simulink model "MIL4L3_SW6_V1_20220211"  (R2018b)
settings: Solver=FixedStepAuto  StartTime=0.0  StopTime=inf  FixedStep=0.001  RelTol=1e-3
PreLoadFcn:
  | A0_MILtest;
undefined symbols (not defined in the file or in its folder): Clb_ICADirect_LaneDisp_StateFive, Clb_ICADirect_LaneDisp_StateFour, Clb_ICADirect_LaneDisp_StateOne, Clb_ICADirect_LaneDisp_StateThree, Clb_ICADirect_LaneDisp_StateTwo, Clb_ICADirect_LaneDisp_StateZero, Clb_ICADirect_LaneDispSW, Clb_ICADirect_TrnLghtsCom_Switch, Clb_ICADirect_TrnLghtsCom_Value, Clb_ICADirect_TrnLghtsCrtl_Inhb, IMAP_Clb_ACU_Driver_Belt, IMAP_Clb_ACU_Driver_Belt_Over, IMAP_Clb_ACU_Passenger_Belt, IMAP_Clb_ACU_Passenger_Belt_Over, IMAP_Clb_ACU_RearLeft_Belt, IMAP_Clb_ACU_RearLeft_Belt_Over, IMAP_Clb_ACU_RearMiddle_Belt, IMAP_Clb_ACU_RearMiddle_Belt_Over, IMAP_Clb_ACU_RearRight_Belt, IMAP_Clb_ACU_RearRight_Belt_Over, IMAP_Clb_AEB_Switch, IMAP_Clb_AEB_Switch_Over, IMAP_Clb_ALC_TLC_Mode, IMAP_Clb_ALC_TLC_Mode_Over, IMAP_Clb_BCM_Battery_Voltage, IMAP_Clb_BCM_Battery_Voltage_Over, IMAP_Clb_BCM_BrakeLamp_State, IMAP_Clb_BCM_BrakeLamp_State_Over, IMAP_Clb_BCM_CHMSL_Status, IMAP_Clb_BCM_CHMSL_Status_Over, IMAP_Clb_BCM_Door_Lock_State, IMAP_Clb_BCM_Door_Lock_State_Over, IMAP_Clb_BCM_FrontWiper_State, IMAP_Clb_BCM_FrontWiper_State_Over, IMAP_Clb_BCM_FrontWiper_Switch, IMAP_Clb_BCM_FrontWiper_Switch_Over, IMAP_Clb_BCM_HazardLamp, IMAP_Clb_BCM_HazardLamp_Over, IMAP_Clb_BCM_HazardLamp_Switch, IMAP_Clb_BCM_HazardLamp_Switch_Over, IMAP_Clb_BCM_HighBeam_State, IMAP_Clb_BCM_HighBeam_State_Over, IMAP_Clb_BCM_Ignition_State, IMAP_Clb_BCM_Ignition_State_Over, IMAP_Clb_BCM_IHBC_Enabled, IMAP_Clb_BCM_IHBC_Enabled_Over, IMAP_Clb_BCM_Left_Light, IMAP_Clb_BCM_Left_Light_Over, IMAP_Clb_BCM_LeftTurn_Switch, IMAP_Clb_BCM_LeftTurn_Switch_Over, IMAP_Clb_BCM_LF_Door_State, IMAP_Clb_BCM_LF_Door_State_Over, IMAP_Clb_BCM_LowBeam_State, IMAP_Clb_BCM_LowBeam_State_Over, IMAP_Clb_BCM_LR_Door_State, IMAP_Clb_BCM_LR_Door_State_Over, IMAP_Clb_BCM_RF_Door_State, IMAP_Clb_BCM_RF_Door_State_Over, IMAP_Clb_BCM_Right_Light, IMAP_Clb_BCM_Right_Light_Over ... (+547)
libraries: CarMaker4SL x2153, simulink x292, dspstat3 x3, canmsglib x2, simulink_extras x1
(part 13 of 52)

== system MIL4L3_SW6_V1_20220211/CarMaker/VehicleControl/FunctionDataLog/ICA ==
  Bus Selector : BusSelector  OutputSignals=FDMMve_d_IcaFcnConf,FDMMve_d_SignalTStamp
  Bus Selector1 : BusSelector  OutputSignals=IMAPve_d_RCTA_Swtich,IMAPve_d_DOW_Switch,IMAPve_d_JA_Brake_Switch,IMAPve_d_JA_Alert_Switch,IMAPve_d_EPS_LKA_State,IMAPve_d_EPS_Trq_State,IMAPve_d_SAS_Clb_State,IMAPve_d_SAS_Trim_State,IMAPve_d_EPS_TrqLim_State,IMAPve_g_ESC_LatAcc,IMAPve_d_ESC_LatAcc_Valid,IMAPve_g_ESC_YawRate,IMAPve_g_ESC_VehSpd,IMAPve_g_ESC_LonAcc,IMAPve_d_ESC_LonAcc_Valid,IMAPve_g_ESC_Brake_Press,IMAPve_g_ESC_Static_Slope,IMAPve_g_ESC_DySlope_Accuracy,IMAPve_g_ESC_DySlope,IMAPve_g_SW_Angle_Speed,IMAPve_d_BCM_Trunk_State,IMAPve_d_PEPS_Door_Lock_Req,IMAPve_g_EMS_MinTWhl_Offset,IMAPve_g_EMS_ACC_VirtualPedal,IMAPve_d_EMS_AccPedal_Fault,IMAPve_d_ESC_Veh_Standstill,IMAPve_d_TCU_Actual_Gear,IMAPve_d_BCM_Ignition_State,IMAPve_d_SWS_Failure_Status,IMAPve_d_ESC_OFF,IMAPve_d_ESC_AlarmSig,IMAPve_d_ESC_RR_Wheel_Pulse,IMAPve_d_ESC_AEB_Available,IMAPve_d_ESC_ACC_Active,IMAPve_d_BCM_CHMSL_Status,IMAPve_d_BCM_BrakeLamp_State,IMAPve_d_ACU_Passenger_Belt,IMAPve_d_EPB_Warn_Req,IMAPve_d_EPB_Switch_State,IMAPve_d_ESC_Hold_State,IMAPva_g_ORI_Obj_LongDis,IMAPva_g_ORI_Obj_LAngle,IMAPva_g_ORI_Obj_RAngle,IMAPva_g_ORI_Obj_Width,IMAPva_d_ORI_Obj_ID,IMAPve_g_ORI_L0_C3,IMAPve_g_ORI_L0_C2,IMAPve_g_ORI_L0_C1,IMAPve_g_ORI_L0_C0,IMAPve_d_ORI_L0_Type,IMAPve_g_ORI_L0_VR,IMAPve_g_ORI_L0_W,IMAPve_g_ORI_L1_C3,IMAPve_g_ORI_L1_C2,IMAPve_g_ORI_L1_C1,IMAPve_g_ORI_L1_C0,IMAPve_d_ORI_L1_Type,IMAPve_g_ORI_L1_VR,IMAPve_g_ORI_L1_W,IMAPve_g_ORI_R0_C3,IMAPve_g_ORI_R0_C2,IMAPve_g_ORI_R0_C1,IMAPve_g_ORI_R0_C0,IMAPve_d_ORI_R0_LT,IMAPve_g_ORI_R0_VR,IMAPve_g_ORI_R0_W,IMAPve_g_ORI_R1_C3,IMAPve_g_ORI_R1_C2,IMAPve_d_Sensor_Status,IMAPve_d_RF_Radar_Status,IMAPve_d_LR_Radar_Status,IMAPve_d_RR_Radar_Status,IMAPve_d_Fusion_Status,IMAPve_d_Fusion_Time_Stamp,IMAPve_d_obj_Num,IMAPva_d_obj_id,IMAPva_g_obj_pos_x,IMAPva_g_obj_pos_y,IMAPva_g_obj_vel_x,IMAPva_g_obj_vel_y,IMAPva_g_obj_acc_x,IMAPva_g_obj_acc_y,IMAPva_g_obj_pos_var_x,IMAPva_g_obj_pos_var_y,IMAPva_g_obj_pos_var_xy,IMAPva_g_obj_width,IMAPva_g_obj_length,IMAPva_d_obj_class,IMAPva_d_obj_lane,IMAPva_d_obj_status,IMAPva_d_obj_age,IMAPva_d_obj_TurnLight,IMAPva_d_obj_BrakeLight,IMAPva_d_obj_MotionStatus,IMAPve_d_Road_Type,IMAPve_g_L0_C0,IMAPve_g_L0_C1,IMAPve_g_L0_C2,IMAPve_g_L0_C3,IMAPve_g_L0_VR,IMAPve_d_L0_Q,IMAPve_d_L0_Type,IMAPve_g_L0_W,IMAPve_g_R0_C0,IMAPve_g_R0_C1,IMAPve_g_R0_C2,IMAPve_g_R0_C3,IMAPve_g_R0_VR,IMAPve_d_R0_Q,IMAPve_d_R0_Type,IMAPve_g_R0_W,IMAPve_g_L1_C0,IMAPve_g_L1_C1,IMAPve_g_L1_C2,IMAPve_g_L1_C3,IMAPve_g_L1_VR,IMAPve_d_L1_Q,IMAPve_d_L1_Type,IMAPve_g_L1_W,IMAPve_g_R1_C0,IMAPve_g_R1_C1,IMAPve_g_R1_C2,IMAPve_g_R1_C3,IMAPve_g_R1_VR,IMAPve_d_R1_Q,IMAPve_d_R1_Type,IMAPve_g_R1_W,IMAPve_g_L0_C0_Back,IMAPve_g_L0_C1_Back,IMAPve_g_L0_C2_Back,IMAPve_g_L0_C3_Back,IMAPve_g_L0_Range_Back,IMAPve_g_R0_C0_Back,IMAPve_g_R0_C1_Back,IMAPve_g_R0_C2_Back,IMAPve_g_R0_C3_Back,IMAPve_g_R0_Range_Back,IMAPve_g_L1_C0_Back,IMAPve_g_L1_C1_Back,IMAPve_g_L1_C2_Back,IMAPve_g_L1_C3_Back,IMAPve_g_L1_Range_Back,IMAPve_d_APA_AutoPark_WorkSt
  Bus Selector4 : BusSelector  OutputSignals=IMAPve_d_BCM_RF_Door_State,IMAPve_d_TSR_Sign_Type,IMAPve_g_Camera_Signal_Fault
  BusCreator2 : BusCreator  Inputs=158
  Clock1 : Clock
  Constant : Constant  Value=0  OutDataTypeStr=uint32
  Constant1 : Constant  Value=0  OutDataTypeStr=uint32
  Constant2 : Constant  Value=0  OutDataTypeStr=uint16
  Constant3 : Constant  OutDataTypeStr=uint8
  Constant4 : Constant  Value=0  OutDataTypeStr=uint8
  Constant5 : Constant  OutDataTypeStr=uint8
  Constant6 : Constant  Value=0  OutDataTypeStr=uint8
  Data Type Conversion{5..8} (4 alike) : DataTypeConversion
  Read CM Dict4 : CarMaker4SL/Read CM Dict  xname=User.IO.Out.VR_RR  xsync=off
  Read CM Dict5 : CarMaker4SL/Read CM Dict  xname=User.IO.Out.VR_R  xsync=off
  Read CM Dict6 : CarMaker4SL/Read CM Dict  xname=User.IO.Out.VR_LL  xsync=off
  Read CM Dict7 : CarMaker4SL/Read CM Dict  xname=User.IO.Out.VR_L  xsync=off
  Switch{4..7} (4 alike) : Switch  Threshold=20
  To Workspace : ToWorkspace  VariableName=ICABIn  SaveFormat=Timeseries  SampleTime=-1
  wires:
  Switch7/1 -> BusCreator2/100  "IMAPve_g_L0_VR"
  [ACCSva_d_ACCS2ICAB] -> BusCreator2/2  "ACCSva_d_ACCS2ICA"
  [EPS_LKA_State_ica] -> BusCreator2/5  "EPS_LKA_State"
  Clock1/1 -> BusCreator2/1  "System_Clock"
  BusCreator2/1 -> To Workspace/1
  Constant1/1 -> BusCreator2/150  "ADIAve_g_BSWFaultStatus"
  Constant/1 -> BusCreator2/149  "ADIAve_g_ASWFaultStatus"
  Constant3/1 -> BusCreator2/152  "EWWWve_y_BSD_LCWWorkingSt"
  Constant2/1 -> BusCreator2/151  "ADIAve_d_FuncFaultStatus"
  Constant6/1 -> BusCreator2/155  "EWWWve_y_BSD_S_LCAWarning"
  Constant4/1 -> BusCreator2/153  "EWWWve_y_BSD_LCAWarning"
  Constant5/1 -> BusCreator2/154  "EWWWve_y_BSD_S_LCWWorkingSt"
  Bus Selector4/2 -> BusCreator2/157  "<IMAPve_d_TSR_Sign_Type>"
  Bus Selector4/1 -> BusCreator2/156  "<IMAPve_d_BCM_RF_Door_State>"
  Bus Selector4/3 -> BusCreator2/158  "<IMAPve_g_Camera_Signal_Fault>"
  [IMAP_Output] -> Bus Selector1/1, Bus Selector4/1
  Read CM Dict4/1 -> Data Type Conversion8/1
  Bus Selector1/15 -> BusCreator2/20  "<IMAPve_d_ESC_LonAcc_Valid>"
  Bus Selector1/2 -> BusCreator2/7  "<IMAPve_d_DOW_Switch>"
  Bus Selector1/16 -> BusCreator2/21  "<IMAPve_g_ESC_Brake_Press>"
  Bus Selector1/9 -> BusCreator2/14  "<IMAPve_d_EPS_TrqLim_State>"
  Bus Selector1/11 -> BusCreator2/16  "<IMAPve_d_ESC_LatAcc_Valid>"
  Bus Selector1/13 -> BusCreator2/18  "<IMAPve_g_ESC_VehSpd>"
  Switch5/1 -> BusCreator2/108  "IMAPve_g_R0_VR"
  Bus Selector1/7 -> BusCreator2/12  "<IMAPve_d_SAS_Clb_State>"
  Bus Selector1/5 -> BusCreator2/10  "<IMAPve_d_EPS_LKA_State>"
  Bus Selector1/92 -> BusCreator2/97  "<IMAPva_d_obj_TurnLight>"
  Bus Selector1/52 -> BusCreator2/57  "<IMAPve_g_ORI_L0_W>"
  Bus Selector1/140 -> BusCreator2/145  "<IMAPve_g_L1_C2_Back>"
  Bus Selector1/62 -> BusCreator2/67  "<IMAPve_g_ORI_R0_C1>"
  Bus Selector1/115 -> BusCreator2/120  "<IMAPve_g_L1_C3>"
  Bus Selector1/87 -> BusCreator2/92  "<IMAPva_g_obj_length>"
  Bus Selector1/139 -> BusCreator2/144  "<IMAPve_g_L1_C1_Back>"
  Bus Selector1/22 -> BusCreator2/27  "<IMAPve_d_PEPS_Door_Lock_Req>"
  Bus Selector1/136 -> BusCreator2/141  "<IMAPve_g_R0_C3_Back>"
  Bus Selector1/132 -> BusCreator2/137  "<IMAPve_g_L0_Range_Back>"
  Bus Selector1/73 -> BusCreator2/78  "<IMAPve_d_Fusion_Status>"
  Bus Selector1/124 -> BusCreator2/129  "<IMAPve_g_R1_VR>"
  Bus Selector1/38 -> BusCreator2/43  "<IMAPve_d_EPB_Warn_Req>"
  Bus Selector1/122 -> BusCreator2/127  "<IMAPve_g_R1_C2>"
  Bus Selector1/105 -> BusCreator2/110  "<IMAPve_g_R0_C1>"
  Bus Selector1/137 -> BusCreator2/142  "<IMAPve_g_R0_Range_Back>"
  Bus Selector1/34 -> BusCreator2/39  "<IMAPve_d_ESC_ACC_Active>"
  Bus Selector1/133 -> BusCreator2/138  "<IMAPve_g_R0_C0_Back>"
  Bus Selector1/129 -> BusCreator2/134  "<IMAPve_g_L0_C1_Back>"
  Bus Selector1/109 -> BusCreator2/114  "<IMAPve_d_R0_Q>"
  Bus Selector1/126 -> BusCreator2/131  "<IMAPve_d_R1_Type>"
  Bus Selector1/56 -> BusCreator2/61  "<IMAPve_g_ORI_L1_C0>"
  Bus Selector1/106 -> BusCreator2/111  "<IMAPve_g_R0_C2>"
  Bus Selector1/93 -> BusCreator2/98  "<IMAPva_d_obj_BrakeLight>"
  Bus Selector1/127 -> BusCreator2/132  "<IMAPve_g_R1_W>"
  Bus Selector1/125 -> BusCreator2/130  "<IMAPve_d_R1_Q>"
  Bus Selector1/123 -> BusCreator2/128  "<IMAPve_g_R1_C3>"
  Bus Selector1/96 -> BusCreator2/101  "<IMAPve_g_L0_C0>"
  Bus Selector1/29 -> BusCreator2/34  "<IMAPve_d_SWS_Failure_Status>"
  Bus Selector1/114 -> BusCreator2/119  "<IMAPve_g_L1_C2>"
  Switch4/1 -> BusCreator2/124  "IMAPve_g_R1_VR"
  Bus Selector1/118 -> BusCreator2/123  "<IMAPve_d_L1_Type>"
  Bus Selector1/97 -> BusCreator2/102  "<IMAPve_g_L0_C1>"
  Bus Selector1/121 -> BusCreator2/126  "<IMAPve_g_R1_C1>"
  Bus Selector1/82 -> BusCreator2/87  "<IMAPva_g_obj_acc_y>"
  Bus Selector1/110 -> BusCreator2/115  "<IMAPve_d_R0_Type>"
  Bus Selector1/113 -> BusCreator2/118  "<IMAPve_g_L1_C1>"
  Bus Selector1/45 -> BusCreator2/50  "<IMAPva_d_ORI_Obj_ID>"
  Bus Selector1/80 -> BusCreator2/85  "<IMAPva_g_obj_vel_y>"
  Bus Selector1/24 -> BusCreator2/29  "<IMAPve_g_EMS_ACC_VirtualPedal>"
  Bus Selector1/117 -> BusCreator2/122  "<IMAPve_d_L1_Q>"
  Bus Selector1/128 -> BusCreator2/133  "<IMAPve_g_L0_C0_Back>"
  Bus Selector1/108 -> BusCreator2/113  "<IMAPve_g_R0_VR>"
  Bus Selector1/112 -> BusCreator2/117  "<IMAPve_g_L1_C0>"
  Bus Selector1/99 -> BusCreator2/104  "<IMAPve_g_L0_C3>"
  Bus Selector1/100 -> BusCreator2/105  "<IMAPve_g_L0_VR>"
  Bus Selector1/107 -> BusCreator2/112  "<IMAPve_g_R0_C3>"
  Bus Selector1/88 -> BusCreator2/93  "<IMAPva_d_obj_class>"
  Bus Selector1/102 -> BusCreator2/107  "<IMAPve_d_L0_Type>"
  Bus Selector1/101 -> BusCreator2/106  "<IMAPve_d_L0_Q>"
  Data Type Conversion6/1 -> Switch5/2, Switch5/3
  Bus Selector1/79 -> BusCreator2/84  "<IMAPva_g_obj_vel_x>"
  Bus Selector1/98 -> BusCreator2/103  "<IMAPve_g_L0_C2>"
  Bus Selector1/86 -> BusCreator2/91  "<IMAPva_g_obj_width>"
  Bus Selector1/17 -> BusCreator2/22  "<IMAPve_g_ESC_Static_Slope>"
  Bus Selector1/81 -> BusCreator2/86  "<IMAPva_g_obj_acc_x>"
  Bus Selector1/23 -> BusCreator2/28  "<IMAPve_g_EMS_MinTWhl_Offset>"
  Bus Selector1/77 -> BusCreator2/82  "<IMAPva_g_obj_pos_x>"
  Bus Selector1/59 -> BusCreator2/64  "<IMAPve_g_ORI_L1_W>"
  Bus Selector1/85 -> BusCreator2/90  "<IMAPva_g_obj_pos_var_xy>"
  Bus Selector1/95 -> Switch7/1  "<IMAPve_d_Road_Type>"
  Bus Selector1/84 -> BusCreator2/89  "<IMAPva_g_obj_pos_var_y>"
  Bus Selector1/91 -> BusCreator2/96  "<IMAPva_d_obj_age>"
  Bus Selector1/83 -> BusCreator2/88  "<IMAPva_g_obj_pos_var_x>"
  Bus Selector1/21 -> BusCreator2/26  "<IMAPve_d_BCM_Trunk_State>"
  Bus Selector1/27 -> BusCreator2/32  "<IMAPve_d_TCU_Actual_Gear>"
  Bus Selector1/135 -> BusCreator2/140  "<IMAPve_g_R0_C2_Back>"
  Bus Selector1/57 -> BusCreator2/62  "<IMAPve_d_ORI_L1_Type>"
  Bus Selector1/138 -> BusCreator2/143  "<IMAPve_g_L1_C0_Back>"
  Bus Selector1/14 -> BusCreator2/19  "<IMAPve_g_ESC_LonAcc>"
  Bus Selector1/12 -> BusCreator2/17  "<IMAPve_g_ESC_YawRate>"
  Bus Selector1/72 -> BusCreator2/77  "<IMAPve_d_RR_Radar_Status>"
  Bus Selector1/36 -> BusCreator2/41  "<IMAPve_d_BCM_BrakeLamp_State>"
  Bus Selector1/103 -> Switch5/1  "<IMAPve_g_L0_W>"
  Bus Selector1/70 -> BusCreator2/75  "<IMAPve_d_RF_Radar_Status>"
  Bus Selector1/39 -> BusCreator2/44  "<IMAPve_d_EPB_Switch_State>"
  Bus Selector1/65 -> BusCreator2/70  "<IMAPve_g_ORI_R0_VR>"
  Bus Selector1/61 -> BusCreator2/66  "<IMAPve_g_ORI_R0_C2>"
  Bus Selector1/26 -> BusCreator2/31  "<IMAPve_d_ESC_Veh_Standstill>"
  Bus Selector1/78 -> BusCreator2/83  "<IMAPva_g_obj_pos_y>"
  Bus Selector1/74 -> BusCreator2/79  "<IMAPve_d_Fusion_Time_Stamp>"
  Bus Selector1/64 -> BusCreator2/69  "<IMAPve_d_ORI_R0_LT>"
  Bus Selector1/60 -> BusCreator2/65  "<IMAPve_g_ORI_R0_C3>"
  Bus Selector1/1 -> BusCreator2/6  "<IMAPve_d_RCTA_Swtich>"
  Bus Selector1/58 -> BusCreator2/63  "<IMAPve_g_ORI_L1_VR>"
  Bus Selector1/68 -> BusCreator2/73  "<IMAPve_g_ORI_R1_C2>"
  Bus Selector1/53 -> BusCreator2/58  "<IMAPve_g_ORI_L1_C3>"
  Bus Selector1/10 -> BusCreator2/15  "<IMAPve_g_ESC_LatAcc>"
  Bus Selector1/66 -> BusCreator2/71  "<IMAPve_g_ORI_R0_W>"
  Bus Selector1/30 -> BusCreator2/35  "<IMAPve_d_ESC_OFF>"
  Bus Selector1/47 -> BusCreator2/52  "<IMAPve_g_ORI_L0_C2>"
  Bus Selector1/51 -> BusCreator2/56  "<IMAPve_g_ORI_L0_VR>"
  Bus Selector1/32 -> BusCreator2/37  "<IMAPve_d_ESC_RR_Wheel_Pulse>"
  Bus Selector1/55 -> BusCreator2/60  "<IMAPve_g_ORI_L1_C1>"
  Bus Selector1/54 -> BusCreator2/59  "<IMAPve_g_ORI_L1_C2>"
  Bus Selector1/71 -> BusCreator2/76  "<IMAPve_d_LR_Radar_Status>"
  Bus Selector1/48 -> BusCreator2/53  "<IMAPve_g_ORI_L0_C1>"
  Bus Selector1/63 -> BusCreator2/68  "<IMAPve_g_ORI_R0_C0>"
  Bus Selector1/50 -> BusCreator2/55  "<IMAPve_d_ORI_L0_Type>"
  Bus Selector1/76 -> BusCreator2/81  "<IMAPva_d_obj_id>"
  Bus Selector1/130 -> BusCreator2/135  "<IMAPve_g_L0_C2_Back>"
  Bus Selector1/41 -> BusCreator2/46  "<IMAPva_g_ORI_Obj_LongDis>"
  Bus Selector1/43 -> BusCreator2/48  "<IMAPva_g_ORI_Obj_RAngle>"
  Bus Selector1/42 -> BusCreator2/47  "<IMAPva_g_ORI_Obj_LAngle>"
  Bus Selector1/44 -> BusCreator2/49  "<IMAPva_g_ORI_Obj_Width>"
  Bus Selector1/3 -> BusCreator2/8  "<IMAPve_d_JA_Brake_Switch>"
  Bus Selector1/19 -> BusCreator2/24  "<IMAPve_g_ESC_DySlope>"
  Bus Selector1/20 -> BusCreator2/25  "<IMAPve_g_SW_Angle_Speed>"
  Bus Selector1/67 -> BusCreator2/72  "<IMAPve_g_ORI_R1_C3>"
  Bus Selector1/35 -> BusCreator2/40  "<IMAPve_d_BCM_CHMSL_Status>"
  Switch6/1 -> BusCreator2/116  "IMAPve_g_L1_VR"
  Bus Selector1/40 -> BusCreator2/45  "<IMAPve_d_ESC_Hold_State>"
  Bus Selector1/25 -> BusCreator2/30  "<IMAPve_d_EMS_AccPedal_Fault>"
  Bus Selector1/6 -> BusCreator2/11  "<IMAPve_d_EPS_Trq_State>"
  Data Type Conversion8/1 -> Switch4/3, Switch4/2
  Bus Selector1/33 -> BusCreator2/38  "<IMAPve_d_ESC_AEB_Available>"
  Bus Selector1/75 -> BusCreator2/80  "<IMAPve_d_obj_Num>"
  Bus Selector1/4 -> BusCreator2/9  "<IMAPve_d_JA_Alert_Switch>"
  Read CM Dict5/1 -> Data Type Conversion6/1
  Read CM Dict7/1 -> Data Type Conversion5/1
  Data Type Conversion7/1 -> Switch6/2, Switch6/3
  Bus Selector1/18 -> BusCreator2/23  "<IMAPve_g_ESC_DySlope_Accuracy>"
  Bus Selector1/94 -> BusCreator2/99  "<IMAPva_d_obj_MotionStatus>"
  Read CM Dict6/1 -> Data Type Conversion7/1
  Bus Selector1/49 -> BusCreator2/54  "<IMAPve_g_ORI_L0_C0>"
  Bus Selector1/104 -> BusCreator2/109  "<IMAPve_g_R0_C0>"
  Bus Selector1/131 -> BusCreator2/136  "<IMAPve_g_L0_C3_Back>"
  Data Type Conversion5/1 -> Switch7/3, Switch7/2
  Bus Selector1/46 -> BusCreator2/51  "<IMAPve_g_ORI_L0_C3>"
  Bus Selector1/8 -> BusCreator2/13  "<IMAPve_d_SAS_Trim_State>"
  Bus Selector1/90 -> BusCreator2/95  "<IMAPva_d_obj_status>"
  Bus Selector1/141 -> BusCreator2/146  "<IMAPve_g_L1_C3_Back>"
  Bus Selector1/31 -> BusCreator2/36  "<IMAPve_d_ESC_AlarmSig>"
  Bus Selector1/143 -> BusCreator2/148  "<IMAPve_d_APA_AutoPark_WorkSt>"
  Bus Selector1/28 -> BusCreator2/33  "<IMAPve_d_BCM_Ignition_State>"
  Bus Selector1/37 -> BusCreator2/42  "<IMAPve_d_ACU_Passenger_Belt>"
  Bus Selector1/134 -> BusCreator2/139  "<IMAPve_g_R0_C1_Back>"
  Bus Selector1/69 -> BusCreator2/74  "<IMAPve_d_Sensor_Status>"
  Bus Selector1/120 -> BusCreator2/125  "<IMAPve_g_R1_C0>"
  Bus Selector1/142 -> BusCreator2/147  "<IMAPve_g_L1_Range_Back>"
  Bus Selector1/116 -> BusCreator2/121  "<IMAPve_g_L1_VR>"
  Bus Selector1/89 -> BusCreator2/94  "<IMAPva_d_obj_lane>"
  Bus Selector1/111 -> Switch6/1  "<IMAPve_g_R0_W>"
  Bus Selector1/119 -> Switch4/1  "<IMAPve_g_L1_W>"
  [FDMM_output] -> Bus Selector/1
  Bus Selector/1 -> BusCreator2/3  "<FDMMve_d_IcaFcnConf>"
  Bus Selector/2 -> BusCreator2/4  "<FDMMve_d_SignalTStamp>"

== system MIL4L3_SW6_V1_20220211/CarMaker/VehicleControl/FunctionDataLog/JA ==
  Bus Selector11 : BusSelector  OutputSignals=FDMMve_d_JaFcnConf
  Bus Selector12 : BusSelector  OutputSignals=IMAPve_d_JA_Alert_Switch,IMAPve_d_JA_Brake_Switch,IMAPve_g_ESC_LatAcc,IMAPve_g_ESC_YawRate,IMAPve_d_ESC_YawRate_Valid,IMAPve_g_ESC_VehSpd,IMAPve_g_ESC_LonAcc,IMAPve_d_ESC_LonAcc_Valid,IMAPve_g_ESC_Static_Slope,IMAPve_g_SW_Angle,IMAPve_g_SW_Angle_Speed,IMAPve_d_BCM_HazardLamp,IMAPve_d_BCM_Left_Light,IMAPve_d_BCM_Right_Light,IMAPve_d_BCM_Opening_State,IMAPve_g_EMS_RealPedal,IMAPve_d_ESC_Veh_Standstill,IMAPve_d_BCM_Ignition_State,IMAPve_d_ACU_Driver_Belt,IMAPve_d_SWS_Failure_Status,IMAPve_d_ESC_OFF,IMAPve_d_ESC_AlarmSig,IMAPve_d_ESC_ESC_Active,IMAPve_d_ESC_VehSpd_Valid,IMAPve_d_ESC_ABS_Active,IMAPve_d_ESC_FL_WheelPulVal,IMAPve_d_ESC_FR_WheelPulVal,IMAPve_d_ESC_RL_WheelPulVal,IMAPve_d_ESC_RR_WheelPulVal,IMAPve_d_TCU_AT_Failure,IMAPve_d_EMS_Engine_Status,IMAPve_d_ESC_AEB_Available,IMAPve_d_ESC_AEB_Active,IMAPve_d_BCM_FrontWiper_State,IMAPve_d_BCM_CHMSL_Status,IMAPve_d_BCM_BrakeLamp_State,IMAPve_d_ACU_Passenger_Belt,IMAPve_d_EMS_Brake_Pedal,IMAPve_d_EPB_Status,IMAPve_d_ESC_Drive_Direction,IMAPve_d_ESC_Hold_State,IMAPve_d_Sensor_Status,IMAPve_d_LF_Radar_Status,IMAPve_d_RF_Radar_Status,IMAPve_d_LR_Radar_Status,IMAPve_d_RR_Radar_Status,IMAPve_d_Fusion_Status,IMAPve_d_obj_Num,IMAPva_d_obj_id,IMAPva_g_obj_pos_x,IMAPva_g_obj_pos_y,IMAPva_g_obj_vel_x,IMAPva_g_obj_vel_y,IMAPva_g_obj_acc_x,IMAPva_g_obj_acc_y,IMAPva_g_obj_pos_var_x,IMAPva_g_obj_pos_var_y,IMAPva_g_obj_pos_var_xy,IMAPva_g_obj_width,IMAPva_g_obj_length,IMAPva_d_obj_class,IMAPva_d_obj_lane,IMAPva_d_obj_status,IMAPva_d_obj_age,IMAPva_d_obj_TurnLight,IMAPva_d_obj_BrakeLight,IMAPva_d_obj_MotionStatus,IMAPve_g_Camera_Signal_Fault,IMAPve_d_Camera_Status,IMAPve_d_ORI_CIPV_ID,IMAPve_d_ORI_Obj_Num,IMAPva_d_ORI_Obj_Class,IMAPva_g_ORI_Obj_RelVel,IMAPva_g_ORI_Obj_LongDis,IMAPva_g_ORI_Obj_LAngle,IMAPva_g_ORI_Obj_RAngle,IMAPva_g_ORI_Obj_Width,IMAPva_d_ORI_Obj_ID
  Bus Selector13 : BusSelector  OutputSignals=IMAPve_d_BCM_HazardLamp_Switch,IMAPve_d_ESC_MSR_Active,IMAPve_d_ESC_TCS_Active
  Bus Selector14 : BusSelector  OutputSignals=IMAPve_d_APA_AutoPark_WorkSt,IMAPve_d_EPS_Warning_State,IMAPve_d_BCM_LeftTurn_Switch,IMAPve_d_BCM_RightTurn_Switch,IMAPve_d_Radar_State,IMAPve_d_Camera_State
  Bus Selector15 : BusSelector  OutputSignals=IMAPve_d_EPS_Trq_State,IMAPve_g_EPS_SW_Trq
  BusCreator : BusCreator  Inputs=95
  Delay : Delay  DelayLength=1
  To Workspace : ToWorkspace  VariableName=JA_Input  SaveFormat=Timeseries  SampleTime=-1
  wires:
  Bus Selector12/60 -> BusCreator/61  "<IMAPva_g_obj_length>"
  Bus Selector12/63 -> BusCreator/64  "<IMAPva_d_obj_status>"
  Bus Selector12/65 -> BusCreator/66  "<IMAPva_d_obj_TurnLight>"
  Bus Selector12/64 -> BusCreator/65  "<IMAPva_d_obj_age>"
  Bus Selector13/2 -> BusCreator/94  "<IMAPve_d_ESC_MSR_Active>"
  Bus Selector12/74 -> BusCreator/75  "<IMAPva_g_ORI_Obj_LongDis>"
  Bus Selector14/2 -> BusCreator/82  "<IMAPve_d_EPS_Warning_State>"
  Bus Selector13/3 -> BusCreator/95  "<IMAPve_d_ESC_TCS_Active>"
  Bus Selector12/28 -> BusCreator/29  "<IMAPve_d_ESC_RL_WheelPulVal>"
  Bus Selector12/16 -> BusCreator/17  "<IMAPve_g_EMS_RealPedal>"
  Bus Selector12/68 -> BusCreator/69  "<IMAPve_g_Camera_Signal_Fault>"
  Bus Selector12/43 -> BusCreator/44  "<IMAPve_d_LF_Radar_Status>"
  Bus Selector15/2 -> BusCreator/89  "<IMAPve_g_EPS_SW_Trq>"
  Bus Selector13/1 -> BusCreator/93  "<IMAPve_d_BCM_HazardLamp_Switch>"
  Bus Selector12/50 -> BusCreator/51  "<IMAPva_g_obj_pos_x>"
  Bus Selector12/70 -> BusCreator/71  "<IMAPve_d_ORI_CIPV_ID>"
  Bus Selector12/67 -> BusCreator/68  "<IMAPva_d_obj_MotionStatus>"
  Bus Selector14/3 -> BusCreator/83  "<IMAPve_d_BCM_LeftTurn_Switch>"
  Bus Selector14/6 -> BusCreator/86  "<IMAPve_d_Camera_State>"
  Bus Selector12/3 -> BusCreator/4  "<IMAPve_g_ESC_LatAcc>"
  Bus Selector12/66 -> BusCreator/67  "<IMAPva_d_obj_BrakeLight>"
  Bus Selector12/73 -> BusCreator/74  "<IMAPva_g_ORI_Obj_RelVel>"
  Bus Selector12/45 -> BusCreator/46  "<IMAPve_d_LR_Radar_Status>"
  Bus Selector12/76 -> BusCreator/77  "<IMAPva_g_ORI_Obj_RAngle>"
  Bus Selector12/23 -> BusCreator/24  "<IMAPve_d_ESC_ESC_Active>"
  Bus Selector12/31 -> BusCreator/32  "<IMAPve_d_EMS_Engine_Status>"
  Bus Selector12/26 -> BusCreator/27  "<IMAPve_d_ESC_FL_WheelPulVal>"
  Bus Selector12/69 -> BusCreator/70  "<IMAPve_d_Camera_Status>"
  Bus Selector12/9 -> BusCreator/10  "<IMAPve_g_ESC_Static_Slope>"
  Bus Selector12/75 -> BusCreator/76  "<IMAPva_g_ORI_Obj_LAngle>"
  Bus Selector12/77 -> BusCreator/78  "<IMAPva_g_ORI_Obj_Width>"
  Bus Selector12/35 -> BusCreator/36  "<IMAPve_d_BCM_CHMSL_Status>"
  Bus Selector12/17 -> BusCreator/18  "<IMAPve_d_ESC_Veh_Standstill>"
  Bus Selector12/12 -> BusCreator/13  "<IMAPve_d_BCM_HazardLamp>"
  Bus Selector12/48 -> BusCreator/49  "<IMAPve_d_obj_Num>"
  Bus Selector11/1 -> BusCreator/1  "<FDMMve_d_JaFcnConf>"
  Bus Selector12/58 -> BusCreator/59  "<IMAPva_g_obj_pos_var_xy>"
  Bus Selector12/40 -> BusCreator/41  "<IMAPve_d_ESC_Drive_Direction>"
  Bus Selector12/39 -> BusCreator/40  "<IMAPve_d_EPB_Status>"
  Bus Selector12/42 -> BusCreator/43  "<IMAPve_d_Sensor_Status>"
  Bus Selector12/41 -> BusCreator/42  "<IMAPve_d_ESC_Hold_State>"
  Bus Selector12/36 -> BusCreator/37  "<IMAPve_d_BCM_BrakeLamp_State>"
  Bus Selector12/37 -> BusCreator/38  "<IMAPve_d_ACU_Passenger_Belt>"
  Bus Selector12/38 -> BusCreator/39  "<IMAPve_d_EMS_Brake_Pedal>"
  Bus Selector12/8 -> BusCreator/9  "<IMAPve_d_ESC_LonAcc_Valid>"
  Bus Selector12/25 -> BusCreator/26  "<IMAPve_d_ESC_ABS_Active>"
  Bus Selector12/32 -> BusCreator/33  "<IMAPve_d_ESC_AEB_Available>"
  [IMAP_Output] -> Bus Selector12/1, Bus Selector13/1, Bus Selector15/1, Bus Selector14/1
  Bus Selector12/22 -> BusCreator/23  "<IMAPve_d_ESC_AlarmSig>"
  Bus Selector12/33 -> BusCreator/34  "<IMAPve_d_ESC_AEB_Active>"
  Bus Selector15/1 -> BusCreator/88  "<IMAPve_d_EPS_Trq_State>"
  Bus Selector12/19 -> BusCreator/20  "<IMAPve_d_ACU_Driver_Belt>"
  Bus Selector12/24 -> BusCreator/25  "<IMAPve_d_ESC_VehSpd_Valid>"
  Bus Selector12/20 -> BusCreator/21  "<IMAPve_d_SWS_Failure_Status>"
  Bus Selector12/18 -> BusCreator/19  "<IMAPve_d_BCM_Ignition_State>"
  Bus Selector12/34 -> BusCreator/35  "<IMAPve_d_BCM_FrontWiper_State>"
  Bus Selector12/14 -> BusCreator/15  "<IMAPve_d_BCM_Right_Light>"
  Bus Selector12/2 -> BusCreator/3  "<IMAPve_d_JA_Brake_Switch>"
  Bus Selector12/29 -> BusCreator/30  "<IMAPve_d_ESC_RR_WheelPulVal>"
  Bus Selector12/11 -> BusCreator/12  "<IMAPve_g_SW_Angle_Speed>"
  Bus Selector12/15 -> BusCreator/16  "<IMAPve_d_BCM_Opening_State>"
  Bus Selector12/21 -> BusCreator/22  "<IMAPve_d_ESC_OFF>"
  Bus Selector12/6 -> BusCreator/7  "<IMAPve_g_ESC_VehSpd>"
  Bus Selector12/7 -> BusCreator/8  "<IMAPve_g_ESC_LonAcc>"
  Bus Selector12/59 -> BusCreator/60  "<IMAPva_g_obj_width>"
  [MDD_deceleration_type] -> BusCreator/80  "ADAS_deceleration_type"
  Bus Selector12/5 -> BusCreator/6  "<IMAPve_d_ESC_YawRate_Valid>"
  Bus Selector12/72 -> BusCreator/73  "<IMAPva_d_ORI_Obj_Class>"
  Bus Selector12/62 -> BusCreator/63  "<IMAPva_d_obj_lane>"
  Bus Selector14/5 -> BusCreator/85  "<IMAPve_d_Radar_State>"
  [ADAS_AEBAlertReq] -> Delay/1
  Bus Selector12/71 -> BusCreator/72  "<IMAPve_d_ORI_Obj_Num>"
  Bus Selector12/1 -> BusCreator/2  "<IMAPve_d_JA_Alert_Switch>"
  Bus Selector12/57 -> BusCreator/58  "<IMAPva_g_obj_pos_var_y>"
  [FDMM_output] -> Bus Selector11/1
  Bus Selector12/46 -> BusCreator/47  "<IMAPve_d_RR_Radar_Status>"
  Bus Selector12/30 -> BusCreator/31  "<IMAPve_d_TCU_AT_Failure>"
  Bus Selector12/54 -> BusCreator/55  "<IMAPva_g_obj_acc_x>"
  Bus Selector14/1 -> BusCreator/81  "<IMAPve_d_APA_AutoPark_WorkSt>"
  Bus Selector12/56 -> BusCreator/57  "<IMAPva_g_obj_pos_var_x>"
  Bus Selector14/4 -> BusCreator/84  "<IMAPve_d_BCM_RightTurn_Switch>"
  Bus Selector12/52 -> BusCreator/53  "<IMAPva_g_obj_vel_x>"
  Bus Selector12/53 -> BusCreator/54  "<IMAPva_g_obj_vel_y>"
  Bus Selector12/55 -> BusCreator/56  "<IMAPva_g_obj_acc_y>"
  Bus Selector12/47 -> BusCreator/48  "<IMAPve_d_Fusion_Status>"
  Bus Selector12/4 -> BusCreator/5  "<IMAPve_g_ESC_YawRate>"
  Bus Selector12/10 -> BusCreator/11  "<IMAPve_g_SW_Angle>"
  Bus Selector12/51 -> BusCreator/52  "<IMAPva_g_obj_pos_y>"
  Bus Selector12/61 -> BusCreator/62  "<IMAPva_d_obj_class>"
  Bus Selector12/44 -> BusCreator/45  "<IMAPve_d_RF_Radar_Status>"
  Delay/1 -> BusCreator/87
  Bus Selector12/49 -> BusCreator/50  "<IMAPva_d_obj_id>"
  Bus Selector12/13 -> BusCreator/14  "<IMAPve_d_BCM_Left_Light>"
  Bus Selector12/78 -> BusCreator/79  "<IMAPva_d_ORI_Obj_ID>"
  Bus Selector12/27 -> BusCreator/28  "<IMAPve_d_ESC_FR_WheelPulVal>"
  BusCreator/1 -> To Workspace/1

== system MIL4L3_SW6_V1_20220211/CarMaker/VehicleControl/FunctionDataLog/LKA ==
  Bus Selector : BusSelector  OutputSignals=IMAPve_d_LKA_Main_Switch,IMAPve_d_LKA_Mode,IMAPve_d_LDW_Warn_Mode,IMAPve_d_APA_AutoPark_WorkSt,IMAPve_d_MP5_Work_State,IMAPve_d_EPS_LKA_State,IMAPve_g_EPS_SW_Trq,IMAPve_d_EPS_Trq_State,IMAPve_d_SAS_Clb_State,IMAPve_d_SAS_Trim_State,IMAPve_d_SWS_Failure_Status,IMAPve_d_EPS_TrqLim_State,IMAPve_g_EPS_LKA_Current,IMAPve_d_EPS_Steer_Hold_State,IMAPve_d_EPS_Driver_Override,IMAPve_d_EPS_ESA_State,IMAPve_d_EPS_SteeringAngle_Flag,IMAPve_g_EPS_SteeringAngle,IMAPve_g_SW_Angle,IMAPve_g_SW_Angle_Speed,IMAPve_g_ESC_LatAcc,IMAPve_d_ESC_LatAcc_Valid,IMAPve_g_ESC_YawRate,IMAPve_d_ESC_YawRate_Valid,IMAPve_g_ESC_UnYawRate,IMAPve_g_ESC_VehSpd,IMAPve_g_ESC_LonAcc,IMAPve_d_ESC_LonAcc_Valid,IMAPve_g_ESC_Brake_Press,IMAPve_d_ESC_VehSpd_Valid,IMAPve_d_BCM_HazardLamp,IMAPve_d_BCM_Left_Light,IMAPve_d_BCM_Right_Light,IMAPve_d_BCM_LeftTurn_Switch,IMAPve_d_BCM_RightTurn_Switch,IMAPve_d_BCM_HazardLamp_Switch,IMAPve_g_EMS_RealPedal,IMAPve_d_TCU_Actual_Gear,IMAPve_d_TCU_TCU_Available
  Bus Selector1 : BusSelector  OutputSignals=FDMMve_d_LkaFcnConf
  Bus Selector2 : BusSelector  OutputSignals=IMAPve_d_Camera_Status,IMAPve_d_Sensor_Status,IMAPve_d_Fusion_Status,IMAPve_g_L0_C0,IMAPve_g_L0_C1,IMAPve_g_L0_C2,IMAPve_g_L0_C3,IMAPve_g_L0_VR,IMAPve_d_L0_Q,IMAPve_d_L0_Type,IMAPve_g_L0_W,IMAPve_g_R0_C0,IMAPve_g_R0_C1,IMAPve_g_R0_C2,IMAPve_g_R0_C3,IMAPve_g_R0_VR,IMAPve_d_R0_Q,IMAPve_d_R0_Type,IMAPve_g_R0_W,IMAPve_g_L1_C0,IMAPve_g_L1_C1,IMAPve_g_L1_C2,IMAPve_g_L1_C3,IMAPve_g_L1_VR,IMAPve_d_L1_Q,IMAPve_d_L1_Type,IMAPve_g_L1_W,IMAPve_g_R1_C0,IMAPve_g_R1_C1,IMAPve_g_R1_C2,IMAPve_g_R1_C3,IMAPve_g_R1_VR,IMAPve_d_R1_Q,IMAPve_d_R1_Type,IMAPve_g_R1_W
  BusCreator : BusCreator  Inputs=78
  To Workspace : ToWorkspace  VariableName=LKA_Input  SaveFormat=Timeseries  SampleTime=-1
  wires:
  ? -> BusCreator/41
  ? -> BusCreator/42
  ? -> BusCreator/43
  Bus Selector/31 -> BusCreator/32  "<IMAPve_d_BCM_HazardLamp>"
  Bus Selector2/31 -> BusCreator/74  "<IMAPve_g_R1_C3>"
  Bus Selector2/23 -> BusCreator/66  "<IMAPve_g_L1_C3>"
  Bus Selector2/33 -> BusCreator/76  "<IMAPve_d_R1_Q>"
  Bus Selector2/7 -> BusCreator/50  "<IMAPve_g_L0_C3>"
  Bus Selector/23 -> BusCreator/24  "<IMAPve_g_ESC_YawRate>"
  Bus Selector/36 -> BusCreator/37  "<IMAPve_d_BCM_HazardLamp_Switch>"
  Bus Selector2/34 -> BusCreator/77  "<IMAPve_d_R1_Type>"
  Bus Selector2/25 -> BusCreator/68  "<IMAPve_d_L1_Q>"
  Bus Selector2/29 -> BusCreator/72  "<IMAPve_g_R1_C1>"
  Bus Selector2/18 -> BusCreator/61  "<IMAPve_d_R0_Type>"
  Bus Selector1/1 -> BusCreator/1  "<FDMMve_d_LkaFcnConf>"
  Bus Selector2/35 -> BusCreator/78  "<IMAPve_g_R1_W>"
  Bus Selector2/5 -> BusCreator/48  "<IMAPve_g_L0_C1>"
  Bus Selector2/28 -> BusCreator/71  "<IMAPve_g_R1_C0>"
  Bus Selector2/27 -> BusCreator/70  "<IMAPve_g_L1_W>"
  Bus Selector2/10 -> BusCreator/53  "<IMAPve_d_L0_Type>"
  Bus Selector2/32 -> BusCreator/75  "<IMAPve_g_R1_VR>"
  Bus Selector2/17 -> BusCreator/60  "<IMAPve_d_R0_Q>"
  Bus Selector2/15 -> BusCreator/58  "<IMAPve_g_R0_C3>"
  Bus Selector/38 -> BusCreator/39  "<IMAPve_d_TCU_Actual_Gear>"
  Bus Selector2/20 -> BusCreator/63  "<IMAPve_g_L1_C0>"
  Bus Selector/4 -> BusCreator/5  "<IMAPve_d_APA_AutoPark_WorkSt>"
  Bus Selector2/13 -> BusCreator/56  "<IMAPve_g_R0_C1>"
  Bus Selector2/26 -> BusCreator/69  "<IMAPve_d_L1_Type>"
  Bus Selector/3 -> BusCreator/4  "<IMAPve_d_LDW_Warn_Mode>"
  Bus Selector2/12 -> BusCreator/55  "<IMAPve_g_R0_C0>"
  Bus Selector2/19 -> BusCreator/62  "<IMAPve_g_R0_W>"
  Bus Selector2/11 -> BusCreator/54  "<IMAPve_g_L0_W>"
  Bus Selector2/4 -> BusCreator/47  "<IMAPve_g_L0_C0>"
  Bus Selector/30 -> BusCreator/31  "<IMAPve_d_ESC_VehSpd_Valid>"
  Bus Selector2/9 -> BusCreator/52  "<IMAPve_d_L0_Q>"
  Bus Selector2/21 -> BusCreator/64  "<IMAPve_g_L1_C1>"
  Bus Selector/39 -> BusCreator/40  "<IMAPve_d_TCU_TCU_Available>"
  Bus Selector/32 -> BusCreator/33  "<IMAPve_d_BCM_Left_Light>"
  Bus Selector/37 -> BusCreator/38  "<IMAPve_g_EMS_RealPedal>"
  Bus Selector2/16 -> BusCreator/59  "<IMAPve_g_R0_VR>"
  Bus Selector/20 -> BusCreator/21  "<IMAPve_g_SW_Angle_Speed>"
  Bus Selector/13 -> BusCreator/14  "<IMAPve_g_EPS_LKA_Current>"
  Bus Selector2/2 -> BusCreator/45  "<IMAPve_d_Sensor_Status>"
  Bus Selector/24 -> BusCreator/25  "<IMAPve_d_ESC_YawRate_Valid>"
  Bus Selector/22 -> BusCreator/23  "<IMAPve_d_ESC_LatAcc_Valid>"
  Bus Selector2/30 -> BusCreator/73  "<IMAPve_g_R1_C2>"
  Bus Selector/6 -> BusCreator/7  "<IMAPve_d_EPS_LKA_State>"
  Bus Selector/28 -> BusCreator/29  "<IMAPve_d_ESC_LonAcc_Valid>"
  Bus Selector/35 -> BusCreator/36  "<IMAPve_d_BCM_RightTurn_Switch>"
  Bus Selector/11 -> BusCreator/12  "<IMAPve_d_SWS_Failure_Status>"
  Bus Selector/25 -> BusCreator/26  "<IMAPve_g_ESC_UnYawRate>"
  [IMAP_Output] -> Bus Selector/1, Bus Selector2/1
  Bus Selector2/1 -> BusCreator/44  "<IMAPve_d_Camera_Status>"
  Bus Selector/10 -> BusCreator/11  "<IMAPve_d_SAS_Trim_State>"
  Bus Selector2/8 -> BusCreator/51  "<IMAPve_g_L0_VR>"
  Bus Selector/9 -> BusCreator/10  "<IMAPve_d_SAS_Clb_State>"
  Bus Selector/1 -> BusCreator/2  "<IMAPve_d_LKA_Main_Switch>"
  Bus Selector/29 -> BusCreator/30  "<IMAPve_g_ESC_Brake_Press>"
  Bus Selector2/6 -> BusCreator/49  "<IMAPve_g_L0_C2>"
  Bus Selector/14 -> BusCreator/15  "<IMAPve_d_EPS_Steer_Hold_State>"
  Bus Selector2/14 -> BusCreator/57  "<IMAPve_g_R0_C2>"
  Bus Selector/7 -> BusCreator/8  "<IMAPve_g_EPS_SW_Trq>"
  Bus Selector/26 -> BusCreator/27  "<IMAPve_g_ESC_VehSpd>"
  Bus Selector/8 -> BusCreator/9  "<IMAPve_d_EPS_Trq_State>"
  Bus Selector/15 -> BusCreator/16  "<IMAPve_d_EPS_Driver_Override>"
  Bus Selector/21 -> BusCreator/22  "<IMAPve_g_ESC_LatAcc>"
  Bus Selector2/22 -> BusCreator/65  "<IMAPve_g_L1_C2>"
  Bus Selector/27 -> BusCreator/28  "<IMAPve_g_ESC_LonAcc>"
  Bus Selector/33 -> BusCreator/34  "<IMAPve_d_BCM_Right_Light>"
  Bus Selector/2 -> BusCreator/3  "<IMAPve_d_LKA_Mode>"
  Bus Selector/34 -> BusCreator/35  "<IMAPve_d_BCM_LeftTurn_Switch>"
  Bus Selector2/3 -> BusCreator/46  "<IMAPve_d_Fusion_Status>"
  Bus Selector/12 -> BusCreator/13  "<IMAPve_d_EPS_TrqLim_State>"
  Bus Selector/17 -> BusCreator/18  "<IMAPve_d_EPS_SteeringAngle_Flag>"
  Bus Selector/18 -> BusCreator/19  "<IMAPve_g_EPS_SteeringAngle>"
  Bus Selector2/24 -> BusCreator/67  "<IMAPve_g_L1_VR>"
  Bus Selector/16 -> BusCreator/17  "<IMAPve_d_EPS_ESA_State>"
  [FDMM_output] -> Bus Selector1/1
  Bus Selector/5 -> BusCreator/6  "<IMAPve_d_MP5_Work_State>"
  Bus Selector/19 -> BusCreator/20  "<IMAPve_g_SW_Angle>"
  BusCreator/1 -> To Workspace/1
